simulink subsystem "PvtSubSys_LATC"  (R2020b)
settings: Solver=VariableStepAuto  StartTime=0.0  StopTime=10.0  RelTol=1e-3
values from neighbouring files (symbols this model uses):
  P_Global_CharSpd_ms : value not decoded    [PubParsGlobal.sldd]
  P_Global_SteeringAngleRatio : value not decoded    [PubParsGlobal.sldd]
  P_Global_WheelBase_m : value not decoded    [PubParsGlobal.sldd]
  P_LCS_A0_Dis_BP : value not decoded    [SubMdlDD_LATC.sldd]
  P_LCS_A2_Curve_BP : value not decoded    [SubMdlDD_LATC.sldd]
  P_LCS_A2_LatAcc_BP : value not decoded    [SubMdlDD_LATC.sldd]
  P_LCS_A2_Pretime = 0.075    [SubMdlDD_LATC.sldd]
  P_LCS_A2S_FliterTime = 0.5    [SubMdlDD_LATC.sldd]
  P_LCS_AngErrReversSign_SourceSW = 1.0    [SubMdlDD_LATC.sldd]
  P_LCS_AngleErrorReversTorq : value not decoded    [SubMdlDD_LATC.sldd]
  P_LCS_AngleErrorReversTorq_LC_TarAngleBp : value not decoded    [SubMdlDD_LATC.sldd]
  P_LCS_AngleErrorReversTorq_LC_TarAngleFac : value not decoded    [SubMdlDD_LATC.sldd]
  P_LCS_AngleErrorReversTorq_LC_VehSpdBp : value not decoded    [SubMdlDD_LATC.sldd]
  P_LCS_AngleErrorReversTorq_LC_VehSpdVal : value not decoded    [SubMdlDD_LATC.sldd]
  P_LCS_AngleErrorReversTorq_VehSpdBp : value not decoded    [SubMdlDD_LATC.sldd]
  P_LCS_AngleErrorReversTorq_VehSpdFac : value not decoded    [SubMdlDD_LATC.sldd]
  P_LCS_AngleFilterTime = 0.1    [SubMdlDD_LATC.sldd]
  P_LCS_AngleSlope_AES_Active = 0.4 0.4 0.4 0.35 0.35 0.35 0.35 0.35 0.35 0.3 0.3 0.3 0.3 0.3 0.3 0.3 0.3 0.3 0.3 0.4 0.4 0.4 0.35 0.35 0.35 0.35 0.35 0.35 0.3 0.3 0.3 0.3 0.3 0.3 0.3 0.3 0.3 0.3 0.4 0.4 0.4 0.35 0.35 0.35 0.35 0.35 0.35 0.3 0.3 0.3 0.3 0.3 0.3 0.3 0.3 0.3 0.3 0.4 0.4 0.4 0.35 0.35 0.35 0.35 0.35 0.35 0.3 0.3 0.3 0.3 0.3 0.3 0.3 0.3 0.3 0.3 0.4 0.4 0.4 0.35 0.35 0.35 0.35 0.35 0.35 0.3 0.3 0.3 0.3 0.3 0.3 0.3 0.    [SubMdlDD_LATC.sldd]
  P_LCS_AngleSlope_ESS_Add = 1.0 1.0 1.0 1.0 2.0 2.0 2.0 7.0 7.0 7.0 7.0 7.0 7.0 7.0 7.0 7.0 7.0 7.0 7.0 1.0 1.0 1.0 1.0 2.0 2.0 2.0 7.0 7.0 7.0 7.0 7.0 7.0 7.0 7.0 7.0 7.0 7.0 7.0 1.0 1.0 1.0 1.0 2.0 2.0 2.0 7.0 7.0 7.0 7.0 7.0 7.0 7.0 7.0 7.0 7.0 7.0 7.0 1.0 1.0 1.0 1.0 2.0 2.0 2.0 7.0 7.0 7.0 7.0 7.0 7.0 7.0 7.0 7.0 7.0 7.0 7.0 1.0 1.0 1.0 1.0 7.5 7.5 7.5 7.5 7.5 7.5 7.5 7.5 7.5 7.5 7.5 8.0 8.0 8.0 8.0 1.0 1.0 1.0 1.0 7.5    [SubMdlDD_LATC.sldd]
  P_LCS_AngleSlope_LC_Eco = 0.4 0.4 0.4 0.35 0.35 0.35 0.35 0.35 0.35 0.3 0.3 0.3 0.3 0.3 0.3 0.3 0.3 0.3 0.3 0.4 0.4 0.4 0.35 0.35 0.35 0.35 0.35 0.35 0.3 0.3 0.3 0.3 0.3 0.3 0.3 0.3 0.3 0.3 0.4 0.4 0.4 0.35 0.35 0.35 0.35 0.35 0.35 0.3 0.3 0.3 0.3 0.3 0.3 0.3 0.3 0.3 0.3 0.4 0.4 0.4 0.35 0.35 0.35 0.35 0.35 0.35 0.3 0.3 0.3 0.3 0.3 0.3 0.3 0.3 0.3 0.3 0.4 0.4 0.4 0.35 0.35 0.35 0.35 0.35 0.35 0.3 0.3 0.3 0.3 0.3 0.3 0.3 0.    [SubMdlDD_LATC.sldd]
  P_LCS_AngleSlope_LC_Nomal = 0.4 0.4 0.4 0.35 0.35 0.35 0.35 0.35 0.35 0.3 0.3 0.3 0.3 0.3 0.3 0.3 0.3 0.3 0.3 0.4 0.4 0.4 0.35 0.35 0.35 0.35 0.35 0.35 0.3 0.3 0.3 0.3 0.3 0.3 0.3 0.3 0.3 0.3 0.4 0.4 0.4 0.35 0.35 0.35 0.35 0.35 0.35 0.3 0.3 0.3 0.3 0.3 0.3 0.3 0.3 0.3 0.3 0.4 0.4 0.4 0.35 0.35 0.35 0.35 0.35 0.35 0.3 0.3 0.3 0.3 0.3 0.3 0.3 0.3 0.3 0.3 0.4 0.4 0.4 0.35 0.35 0.35 0.35 0.35 0.35 0.3 0.3 0.3 0.3 0.3 0.3 0.3 0.    [SubMdlDD_LATC.sldd]
  P_LCS_AngleSlope_LC_Sport = 0.4 0.4 0.4 0.35 0.35 0.35 0.35 0.35 0.35 0.3 0.3 0.3 0.3 0.3 0.3 0.3 0.3 0.3 0.3 0.4 0.4 0.4 0.35 0.35 0.35 0.35 0.35 0.35 0.3 0.3 0.3 0.3 0.3 0.3 0.3 0.3 0.3 0.3 0.4 0.4 0.4 0.35 0.35 0.35 0.35 0.35 0.35 0.3 0.3 0.3 0.3 0.3 0.3 0.3 0.3 0.3 0.3 0.4 0.4 0.4 0.35 0.35 0.35 0.35 0.35 0.35 0.3 0.3 0.3 0.3 0.3 0.3 0.3 0.3 0.3 0.3 0.4 0.4 0.4 0.35 0.35 0.35 0.35 0.35 0.35 0.3 0.3 0.3 0.3 0.3 0.3 0.3 0.    [SubMdlDD_LATC.sldd]
  P_LCS_AngleSlope_LCK = 0.4 0.4 0.4 0.4 0.4 0.4 0.4 0.4 0.4 0.4 0.4 0.4 0.4 0.4 0.4 0.4 0.4 0.4 0.4 0.4 0.4 0.4 0.4 0.4 0.4 0.4 0.4 0.4 0.4 0.4 0.4 0.4 0.4 0.4 0.4 0.4 0.4 0.4 0.4 0.4 0.4 0.4 0.4 0.4 0.4 0.4 0.4 0.4 0.4 0.4 0.4 0.4 0.4 0.4 0.4 0.4 0.4 0.4 0.4 0.4 0.4 0.4 0.4 0.4 0.4 0.4 0.4 0.4 0.4 0.4 0.4 0.4 0.4 0.4 0.4 0.4 0.4 0.4 0.4 0.4 0.4 0.4 0.4 0.4 0.4 0.4 0.4 0.4 0.4 0.4 0.4 0.4 0.4 0.4 0.4 0.4 0.4 0.4 0.4 0.4    [SubMdlDD_LATC.sldd]
  P_LCS_AngleSlope_LCKIE = 0.4 0.4 0.4 0.4 0.4 0.4 0.4 0.4 0.4 0.4 0.4 0.4 0.4 0.4 0.4 0.4 0.4 0.4 0.4 0.4 0.4 0.4 0.4 0.4 0.4 0.4 0.4 0.4 0.4 0.4 0.4 0.4 0.4 0.4 0.4 0.4 0.4 0.4 0.4 0.4 0.4 0.4 0.4 0.4 0.4 0.4 0.4 0.4 0.4 0.4 0.4 0.4 0.4 0.4 0.4 0.4 0.4 0.4 0.4 0.4 0.4 0.4 0.4 0.4 0.4 0.4 0.4 0.4 0.4 0.4 0.4 0.4 0.4 0.4 0.4 0.4 0.4 0.4 0.4 0.4 0.4 0.4 0.4 0.4 0.4 0.4 0.4 0.4 0.4 0.4 0.4 0.4 0.4 0.4 0.4 0.4 0.4 0.4 0.4 0.4    [SubMdlDD_LATC.sldd]
  P_LCS_AngleSlope_LKA = 0.2 0.2 0.3 0.4 0.4 0.4 0.4 0.4 0.4 0.4 0.4 0.4 0.4 0.4 0.4 0.4 0.4 0.4 0.4 0.2 0.2 0.3 0.4 0.4 0.4 0.4 0.4 0.4 0.4 0.4 0.4 0.4 0.4 0.4 0.4 0.4 0.4 0.4 0.2 0.2 0.3 0.4 0.4 0.4 0.4 0.4 0.4 0.4 0.4 0.4 0.4 0.4 0.4 0.4 0.4 0.4 0.4 0.2 0.2 0.3 0.4 0.4 0.4 0.4 0.4 0.4 0.4 0.4 0.4 0.4 0.4 0.4 0.4 0.4 0.4 0.4 0.2 0.2 0.3 0.4 0.4 0.4 0.4 0.4 0.4 0.4 0.4 0.4 0.4 0.4 0.4 0.4 0.4 0.4 0.4 0.2 0.2 0.3 0.4 0.4    [SubMdlDD_LATC.sldd]
  P_LCS_AngleSlope_Spd_BP : value not decoded    [SubMdlDD_LATC.sldd]
  P_LCS_CurAngleFiltEnable = 1    [SubMdlDD_LATC.sldd]
  P_LCS_CurAngleFilterFC = 2.0    [SubMdlDD_LATC.sldd]
  P_LCS_CurentOffset_LimitValue = 0.001    [SubMdlDD_LATC.sldd]
  P_LCS_CurOffset_SterAngleSpd_Enable = 0.0    [SubMdlDD_LATC.sldd]
  P_LCS_CurOffset_SterAngleSpd_LimitValue = 6.0    [SubMdlDD_LATC.sldd]
  P_LCS_CurOffset_VehicleSpd_LimitValue = 7.0    [SubMdlDD_LATC.sldd]
  P_LCS_CurOffsetA2_Enable = 0.0    [SubMdlDD_LATC.sldd]
  P_LCS_CurOffsetA2_FliterTime = 0.2    [SubMdlDD_LATC.sldd]
  P_LCS_DeltaEps_SpdBp : value not decoded    [SubMdlDD_LATC.sldd]
  P_LCS_DeltaEps_TimeVal : value not decoded    [SubMdlDD_LATC.sldd]
  P_LCS_DesAngle_DelaySample : value not decoded    [SubMdlDD_LATC.sldd]
  P_LCS_DetNoOverRide_DrvTrq_TH : value not decoded    [SubMdlDD_LATC.sldd]
  P_LCS_DetOverRide_DrvTrq_TH : value not decoded    [SubMdlDD_LATC.sldd]
  P_LCS_EPSNotActiveSpdValue = 3.0    [SubMdlDD_LATC.sldd]
  P_LCS_ESS_AngleSlope_Limit = 2.9    [SubMdlDD_LATC.sldd]
  P_LCS_ESS_LogicTest_Enable = 1.0    [SubMdlDD_LATC.sldd]
  P_LCS_ESS_MaxTorqSlope : value not decoded    [SubMdlDD_LATC.sldd]
  P_LCS_ESS_NotActiveFlgDelayTime = 0.0    [SubMdlDD_LATC.sldd]
  P_LCS_ESS_NotActiveFlgDelayTimeSW = 0.0    [SubMdlDD_LATC.sldd]
  P_LCS_ESS_SteerAngleErr : value not decoded    [SubMdlDD_LATC.sldd]
  P_LCS_ESS_SteerAngleFilterTime = 0.2    [SubMdlDD_LATC.sldd]
  P_LCS_ESS_TarAngleFilterTime = 0.2    [SubMdlDD_LATC.sldd]
  P_LCS_ESSAngleSW2 = 0.0    [SubMdlDD_LATC.sldd]
  P_LCS_ESSOverrideTime1 = 0.06    [SubMdlDD_LATC.sldd]
  P_LCS_ESSOverrideTime2 = 0.06    [SubMdlDD_LATC.sldd]
  P_LCS_ESSOverrideTime3 = 0.06    [SubMdlDD_LATC.sldd]
  P_LCS_ESSOverrideValue1 = 20.0    [SubMdlDD_LATC.sldd]
  P_LCS_ESSOverrideValue2 = 20.0    [SubMdlDD_LATC.sldd]
  P_LCS_FF_A0_Speed_Factor : value not decoded    [SubMdlDD_LATC.sldd]
  P_LCS_FF_A0_Torq : value not decoded    [SubMdlDD_LATC.sldd]
  P_LCS_FF_EnableSpd = 5.0    [SubMdlDD_LATC.sldd]
  P_LCS_FF_LCRevs_SpdBP : value not decoded    [SubMdlDD_LATC.sldd]
  P_LCS_FF_LCRevs_SpdVal : value not decoded    [SubMdlDD_LATC.sldd]
  P_LCS_FF_LCRevs_TimeBP : value not decoded    [SubMdlDD_LATC.sldd]
  P_LCS_FF_LCRevs_TimeFacVal : value not decoded    [SubMdlDD_LATC.sldd]
  P_LCS_FF_Param_CurveBp : value not decoded    [SubMdlDD_LATC.sldd]
  P_LCS_FF_Param_CurveFac : value not decoded    [SubMdlDD_LATC.sldd]
  P_LCS_FF_Speed_Bp : value not decoded    [SubMdlDD_LATC.sldd]
  P_LCS_FF_Speed_Factor : value not decoded    [SubMdlDD_LATC.sldd]
  P_LCS_FF_TarAngleTorq_Bp : value not decoded    [SubMdlDD_LATC.sldd]
  P_LCS_FF_TarAngleTorq_Factor : value not decoded    [SubMdlDD_LATC.sldd]
  P_LCS_FFW_Torq_AngleBp : value not decoded    [SubMdlDD_LATC.sldd]
  P_LCS_FFW_Torq_SpdBp : value not decoded    [SubMdlDD_LATC.sldd]
  P_LCS_FFW_Torq_V71 : value not decoded    [SubMdlDD_LATC.sldd]
  P_LCS_FFWSwitch : value not decoded    [SubMdlDD_LATC.sldd]
  P_LCS_IN_Offset_Test_SW = 0.0    [SubMdlDD_LATC.sldd]
  P_LCS_IN_Offset_Test_Value = 0.0    [SubMdlDD_LATC.sldd]
  P_LCS_LatAcc2CurveSW = 0.0    [SubMdlDD_LATC.sldd]
  P_LCS_LC_Complete_PreDisFac : value not decoded    [SubMdlDD_LATC.sldd]
  P_LCS_LCK_preDis_Nomal : value not decoded    [SubMdlDD_LATC.sldd]
  P_LCS_MaxTorqSlope : value not decoded    [SubMdlDD_LATC.sldd]
  P_LCS_NoOverRideTime_TH_s : value not decoded    [SubMdlDD_LATC.sldd]
  P_LCS_Offset_FliterTime = 2.0    [SubMdlDD_LATC.sldd]
  P_LCS_OverRideDetect_enable : value not decoded    [SubMdlDD_LATC.sldd]
  P_LCS_OverRideTime_TH_s : value not decoded    [SubMdlDD_LATC.sldd]
  P_LCS_PID_A0_BP : value not decoded    [SubMdlDD_LATC.sldd]
  P_LCS_PID_A0_FF_SW = 0.0    [SubMdlDD_LATC.sldd]
  P_LCS_PID_A0_P : value not decoded    [SubMdlDD_LATC.sldd]
  P_LCS_PID_AngErrFacBp : value not decoded    [SubMdlDD_LATC.sldd]
  P_LCS_PID_AngErrFacBp_P : value not decoded    [SubMdlDD_LATC.sldd]
  P_LCS_PID_AngErrFacVal : value not decoded    [SubMdlDD_LATC.sldd]
  P_LCS_PID_AngErrFacVal_P : value not decoded    [SubMdlDD_LATC.sldd]
  P_LCS_PID_DisableKi_CurveVal = 0.003    [SubMdlDD_LATC.sldd]
  P_LCS_PID_DrvTorqFacBp : value not decoded    [SubMdlDD_LATC.sldd]
  P_LCS_PID_DrvTorqFacVal : value not decoded    [SubMdlDD_LATC.sldd]
  P_LCS_PID_Ki_TarAng_ESS : value not decoded    [SubMdlDD_LATC.sldd]
  P_LCS_PID_Kp_TarAng_ESS : value not decoded    [SubMdlDD_LATC.sldd]
  P_LCS_PID_Kp_TarAng_ESS2 : value not decoded    [SubMdlDD_LATC.sldd]
  P_LCS_PID_Kp_TarTorq_ESS : value not decoded    [SubMdlDD_LATC.sldd]
  P_LCS_PID_Param_CurveBp : value not decoded    [SubMdlDD_LATC.sldd]
  P_LCS_PID_Param_CurveFac : value not decoded    [SubMdlDD_LATC.sldd]
  P_LCS_PID_Param_GainSwitch : value not decoded    [SubMdlDD_LATC.sldd]
  P_LCS_PID_Param_Kd : value not decoded    [SubMdlDD_LATC.sldd]
  P_LCS_PID_Param_KdFilterTime : value not decoded    [SubMdlDD_LATC.sldd]
  P_LCS_PID_Param_Ki : value not decoded    [SubMdlDD_LATC.sldd]
  P_LCS_PID_Param_KiFreaseWhenLC_Enable : value not decoded    [SubMdlDD_LATC.sldd]
  P_LCS_PID_Param_Kp : value not decoded    [SubMdlDD_LATC.sldd]
  P_LCS_PID_Param_Speed_Adapt : value not decoded    [SubMdlDD_LATC.sldd]
  P_LCS_PID_Param_Speed_Factor_D : value not decoded    [SubMdlDD_LATC.sldd]
  P_LCS_PID_Param_Speed_Factor_I : value not decoded    [SubMdlDD_LATC.sldd]
  P_LCS_PID_Param_Speed_Factor_P : value not decoded    [SubMdlDD_LATC.sldd]
  P_LCS_PID_Param_SteerWheelAngle_Adapt : value not decoded    [SubMdlDD_LATC.sldd]
  P_LCS_PID_Param_SteerWheelAngle_Factor_D : value not decoded    [SubMdlDD_LATC.sldd]
  P_LCS_PID_Param_SteerWheelAngle_Factor_P : value not decoded    [SubMdlDD_LATC.sldd]
  P_LCS_PID_Param_SteerWheelSpd_Adapt : value not decoded    [SubMdlDD_LATC.sldd]
  P_LCS_PID_Param_SteerWheelSpd_Factor_D : value not decoded    [SubMdlDD_LATC.sldd]
  P_LCS_PID_Param_SteerWheelSpd_Factor_P : value not decoded    [SubMdlDD_LATC.sldd]
  P_LCS_PID_SteerAngSpdLim : value not decoded    [SubMdlDD_LATC.sldd]
  P_LCS_preDis_AES_Fac = 0.0 0.0 0.0 0.0 -0.1 -0.1 -0.1 -0.1 -0.1 -0.1 0.1 0.1 0.1 0.2 0.2 0.2 0.2 0.2 0.2 0.0 0.0 0.0 0.0 -0.1 -0.1 -0.1 -0.1 -0.1 -0.1 0.1 0.1 0.1 0.2 0.2 0.2 0.2 0.2 0.2 0.0 0.0 0.0 0.0 -0.1 -0.1 -0.1 -0.1 -0.1 -0.1 0.1 0.1 0.1 0.2 0.2 0.2 0.2 0.2 0.2 0.0 0.0 0.0 0.0 -0.1 -0.1 -0.1 -0.1 -0.1 -0.1 0.1 0.1 0.1 0.2 0.2 0.2 0.2 0.2 0.2 0.0 0.0 0.0 0.0 -0.1 -0.1 -0.1 -0.1 -0.1 -0.1 0.2 0.2 0.2 0.35 0.35 0.35    [SubMdlDD_LATC.sldd]
  P_LCS_preDis_LC_Eco_Fac = 0.0 0.0 0.0 0.0 0.25 0.3 0.3 0.3 0.35 0.35 0.45 0.45 0.45 0.55 0.55 0.55 0.55 0.55 0.55 0.0 0.0 0.0 0.0 0.25 0.3 0.3 0.3 0.35 0.35 0.45 0.45 0.45 0.55 0.55 0.55 0.55 0.55 0.55 0.0 0.0 0.0 0.0 0.25 0.3 0.3 0.3 0.35 0.35 0.45 0.45 0.45 0.55 0.55 0.55 0.55 0.55 0.55 0.0 0.0 0.0 0.0 0.25 0.3 0.3 0.3 0.35 0.35 0.45 0.45 0.45 0.55 0.55 0.55 0.55 0.55 0.55 0.0 0.0 0.0 0.0 0.25 0.3 0.3 0.3 0.35 0.35 0.55    [SubMdlDD_LATC.sldd]
  P_LCS_preDis_LC_Fac = 0.0 0.0 0.0 0.0 -0.1 -0.1 -0.1 -0.1 -0.1 -0.1 0.1 0.1 0.1 0.2 0.2 0.2 0.2 0.2 0.2 0.0 0.0 0.0 0.0 -0.1 -0.1 -0.1 -0.1 -0.1 -0.1 0.1 0.1 0.1 0.2 0.2 0.2 0.2 0.2 0.2 0.0 0.0 0.0 0.0 -0.1 -0.1 -0.1 -0.1 -0.1 -0.1 0.1 0.1 0.1 0.2 0.2 0.2 0.2 0.2 0.2 0.0 0.0 0.0 0.0 -0.1 -0.1 -0.1 -0.1 -0.1 -0.1 0.1 0.1 0.1 0.2 0.2 0.2 0.2 0.2 0.2 0.0 0.0 0.0 0.0 -0.1 -0.1 -0.1 -0.1 -0.1 -0.1 0.2 0.2 0.2 0.35 0.35 0.35    [SubMdlDD_LATC.sldd]
  P_LCS_preDis_LC_Nomal_Fac = 0.0 0.0 0.0 0.0 -0.1 -0.1 -0.1 -0.1 -0.1 -0.1 0.1 0.1 0.1 0.2 0.2 0.2 0.2 0.2 0.2 0.0 0.0 0.0 0.0 -0.1 -0.1 -0.1 -0.1 -0.1 -0.1 0.1 0.1 0.1 0.2 0.2 0.2 0.2 0.2 0.2 0.0 0.0 0.0 0.0 -0.1 -0.1 -0.1 -0.1 -0.1 -0.1 0.1 0.1 0.1 0.2 0.2 0.2 0.2 0.2 0.2 0.0 0.0 0.0 0.0 -0.1 -0.1 -0.1 -0.1 -0.1 -0.1 0.1 0.1 0.1 0.2 0.2 0.2 0.2 0.2 0.2 0.0 0.0 0.0 0.0 -0.1 -0.1 -0.1 -0.1 -0.1 -0.1 0.2 0.2 0.2 0.35 0.35 0.35    [SubMdlDD_LATC.sldd]
  P_LCS_preDis_LC_Sport_Fac = 0.0 0.0 0.0 0.0 -0.1 -0.1 -0.1 -0.1 -0.1 -0.1 0.1 0.1 0.1 0.2 0.2 0.2 0.2 0.2 0.2 0.0 0.0 0.0 0.0 -0.1 -0.1 -0.1 -0.1 -0.1 -0.1 0.1 0.1 0.1 0.2 0.2 0.2 0.2 0.2 0.2 0.0 0.0 0.0 0.0 -0.1 -0.1 -0.1 -0.1 -0.1 -0.1 0.1 0.1 0.1 0.2 0.2 0.2 0.2 0.2 0.2 0.0 0.0 0.0 0.0 -0.1 -0.1 -0.1 -0.1 -0.1 -0.1 0.1 0.1 0.1 0.2 0.2 0.2 0.2 0.2 0.2 0.0 0.0 0.0 0.0 -0.1 -0.1 -0.1 -0.1 -0.1 -0.1 0.2 0.2 0.2 0.35 0.35 0.35    [SubMdlDD_LATC.sldd]
  P_LCS_preDis_LCK_A2Curve_Fac2 : value not decoded    [SubMdlDD_LATC.sldd]
  ... (+20 more)
undefined symbols (not defined in the file or in its folder): P_LCS_A2_CurrentOffsetFliterTime, P_LCS_AngleSlope_ELK, P_LCS_AngleSlope_ESS, P_LCS_AngleSlope_LC_Cancel, P_LCS_AngleSlope_LCK_Curve_Fac, P_LCS_CurSteerAngleOffsetLimit_Low, P_LCS_CurSteerAngleOffsetLimit_Up, P_LCS_DesLaneA0, P_LCS_DesLaneA1, P_LCS_ESS_preDis_Nomal, P_LCS_ESSAngleSW, P_LCS_ESSAngSlope_SW, P_LCS_LATC_Effect, P_LCS_MinTorqSlope, P_LCS_PID_Param_Kifactor, P_LCS_preDis_ELK_Fac, P_LCS_preDis_ESS_Fac, P_LCS_preDis_LCK_A2Curve_Fac, P_LCS_preDis_LCK_Fac, P_LCS_StateActiv_AngleSlope, P_LCS_StateActiveFlg_BP, P_LCS_TorqSlope_AngleErrorBp, P_LCS_TorqSlope_AngleErrorVal, P_LCS_TorqSlope_AngleSpdBp, P_LCS_TorqSlope_AngleSpdVal, P_LCS_TorqSlope_TorqErrorBp, P_LCS_TorqSlope_TorqErrorVal
libraries: simulink x59
(part 6 of 75)

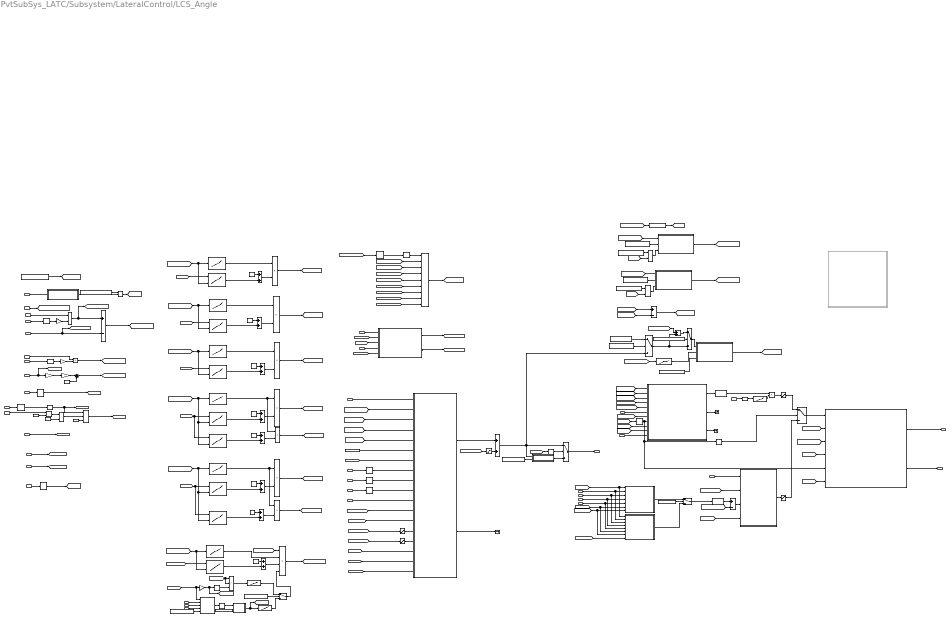
== system PvtSubSys_LATC/Subsystem/LateralControl/LCS_Angle ==
  note: 0:No Function Active
      | 1:LCK Active
      | 2:LCKIE Active
      | 3:LC Normal Active
      | 4:LKA Active
      | 5:ELK Active
      | 6:ESS Active
      | 7:LC Eco Active
      | 8:LC Sport Active
      | 9:LC cancel
      | 10: AES Active
  note: ESS_AES
  note: ELK && LC
  note: Steer Wheel Angle Slope Manage
  note: LCK_LKA_LCKIE_Normal
  note: Sport
  note: Eco
  note: Normal
  note: PreDis_Manage
  note: Torque
  note: 0:No Function Active
      | 1:LCK Active
      | 2:LCKIE Active
      | 3:LC Normal Active
      | 4:LKA Active
      | 5:ELK Active
      | 6:ESS AES Active
      | 7:LC Eco Active
      | 8:LC Sport Active
  note: 模型变更记录
      | 2021/05/31 修改PreDis观测量、增加PreDisFac观测量；（版本：36010506）
      | 2021/06/02 增加弯道关于A2的PreDisFac标定量；（版本：36010506）
      | 2021/06/08 按A0 = 0.8m退出LC修改三种换道预瞄距离系数；增加LCS_EpsTrqReqValue、LCS_EpsTrqReqValueVld观测量（版本：36010506）
      | 2021/06/17 增加单独的ELK、ESSAES预瞄距离参数表；增加LCS_LC_ESSPredis、LCS_LC_ELKPredis观测量；增加ESS、ELS手动调试开关（版本：36170507）
      | 修改LCS模型输出观测量命名，例：LCS_ReqEPSTrgAngle -> LCS_OUT_ReqEPSTrgAngle
      | 2021/07/05 更新ELK标定参数（版本：37050508）
      | 2021/07/12 更新P_LCS_preDis_LCK_A2Curve_Fac标定参数（版本：37120509）
      | 2021/07/15 增加弯道内通过预瞄曲率查表LCK_Predis的Fac修正系数逻辑（版本：37120509）
      | 2021/07/20 增加换道取消P_LCS_preDis_LC_Fac修正系数（版本：37120509）
      | 2021/08/03 增加ESS请求角度斜率限制，防止EPS故障（版本：37120509）
      | 2021/08/04 增加EPS转速>150，ESS退出逻辑，暂用于测试，后期可能会删除（版本：37120509）
      | 2021/08/04 P_LCS_LatAcc2CurveSW设置默认为0
      | 2021/08/09 增加ESS测试逻辑，暂时测试版
      | 2021/08/16 ESS标定数据更改、增加转角与扭矩得ESS开关
      | 2021/08/20 A2项逻辑默认开，LCK_Fac全部置0，P_LCS_preDis_LCK_A2Curve_Fac2参数置：1 1 1 0.85 0.75 0.6 0.5 0.3 0.3 0.25
      | 2021/08/21 修改5kph以下LineValid置零逻辑（版本：38210511）
      | 2021/08/23 修改5kph以下LineValid置零，置零后目标角度不滤波（版本：38210511）
      | 2021/08/23 修改LC换道取消逻辑和标定参数（版本：38230512）
      | 2021/08/24 ESS最初为~=6，因测试出当DangerLevel==6时，状态可能跳变的问题。改成<=5，避免数据类型导致数据比较出现的问题
      | 2021/08/24 增加EPS故障监控逻辑、PID中FF和Kp增加A0项（版本：38240513）
      | 2021/08/25 修改AngleErrorRevers反向符号逻辑（版本：38250514）
      | 2021/08/30 模型整理（版本：38300515）
      | 2021/09/07 修改ESS置位条件（版本：39070516）
      | 2021/09/15 增加port口描述及接口数据类型（版本：39150517）
      | 2021/10/18 LineValid置零逻辑阈值由5kph->3kph;同步CurrentOffset激活逻辑;增加换道超调控制逻辑(默认关闭)（版本：10180518）
      | 2021/10/20 修改内部CurrentOffset激活条件，改成根据曲率进行滤波（版本：10200519)
      | 2021/11/01 增加大框接口LATC_Effect（版本：11010520)
      | 2021/11/03 增加依据曲率修正LCK的AngelSlope（版本：11030521)
      | 2021/11/04 增加内部CurrentOffset计算限值（版本：11040522)
      | 2021/11/08 修改内部CurrentOffset根据曲率进行滤波的时间（版本：11080523)
  note: ESS请求角度斜率限制，防止EPS故障
  note: 最初为~=6，因测试出当DangerLevel==6时，状态可能跳变的问题。改成<=5避免数据类型导致数据比较出现的问题
  canSteerWheelAngle : Inport
  canSteerWheelAngleSign : Inport  Port=2
  canEPS_LKATorqOvrlDlvd : Inport  Port=3
  canEPS_DrvInputTorq : Inport  Port=4
  canSteerWheelSpd : Inport  Port=5
  canSteerWheelSpdSign : Inport  Port=6
  SteerAngleOffset_deg : Inport  Port=7
  eviVxvRef_ms : Inport  Port=8
  desLaneValid : Inport  Port=9
  desLaneA3 : Inport  Port=10  OutDataTypeStr=single
  desLaneA2 : Inport  Port=11
  desLaneA1 : Inport  Port=12
  desLaneA0 : Inport  Port=13
  TarDangerlLevel : Inport  Port=14
  kapTraj1 : Inport  Port=15
  CurrentSteerAngleOffset : Inport  Port=16
  LaneWidth : Inport  Port=17
  2-D Lookup Table1 : Lookup_n-D  BreakpointsForDimension1=P_LCS_A0_Dis_BP  BreakpointsForDimension2=P_LCS_preDis_spd  Table=P_LCS_preDis_LC_Nomal_Fac  ExtrapMethod=Clip  UseLastTableValue=on  InternalRulePriority=Speed  RndMeth=Simplest  InputSameDT=on
      settings: InputPortMap=u0,u1
  2-D Lookup Table2 : Lookup_n-D  BreakpointsForDimension1=P_LCS_A0_Dis_BP  BreakpointsForDimension2=P_LCS_preDis_spd  Table=P_LCS_preDis_LCK_Fac  ExtrapMethod=Clip  UseLastTableValue=on  InternalRulePriority=Speed  RndMeth=Simplest  InputSameDT=on
      settings: InputPortMap=u0,u1
  Abs{1..4} (4 alike) : Abs
  Add : Sum  Inputs=+-
  Add1 : Sum  Inputs=+-
  Add{2,4..5,7..12} (9 alike) : Sum
  Add3 : Sum  Inputs=+-
  Add6 : Sum  AccumDataTypeStr=single
  AngSlopeCalc : Subsystem
  Bias1 : Bias  Bias=-0.5
  Bias2 : Bias  Bias=-0.5
  Compare To Constant : simulink/Logic and Bit Operations/Compare To Constant  relop=~=  const=6  OutDataTypeStr=boolean
  Compare To Constant1 : simulink/Logic and Bit Operations/Compare To Constant  relop=~=  const=6  OutDataTypeStr=boolean
  Compare To Constant3 : simulink/Logic and Bit Operations/Compare To Constant  relop=<=  const=57  OutDataTypeStr=boolean
  Constant : Constant  Value=P_Global_SteeringAngleRatio  OutDataTypeStr=double
  Constant1 : Constant  Value=1000  OutDataTypeStr=single
  Constant10 : Constant  Value=P_LCS_CurAngleFiltEnable
  Constant11 : Constant  Value=P_LCS_TarAngleFilterEnable
  Constant{12..14,17..18,22,24,26} (8 alike) : Constant  OutDataTypeStr=single
  Constant15 : Constant  Value=P_LCS_OverRideDetect_enable
  Constant16 : Constant  Value=P_LCS_ESS_AngleSlope_Limit  OutDataTypeStr=single
  Constant2 : Constant  Value=P_LCS_LatAcc2CurveSW
  Constant20 : Constant  Value=P_LCS_A2S_FliterTime
  Constant21 : Constant  Value=P_LCS_A2_Pretime  OutDataTypeStr=single
  Constant4 : Constant  Value=3.6  OutDataTypeStr=single
  Constant5 : Constant  Value=P_LCS_SW
  Constant6 : Constant  Value=3  OutDataTypeStr=single
  Constant7 : Constant  Value=4  OutDataTypeStr=single
  Constant8 : Constant  Value=1.3  OutDataTypeStr=single
  Constant9 : Constant  Value=P_LCS_CurAngleFiltEnable
  Data Type Conversion : DataTypeConversion  OutDataTypeStr=single
  Data Type Conversion5 : DataTypeConversion  OutDataTypeStr=single
  Direct Lookup Table (n-D) : LookupNDDirect  NumberOfTableDimensions=1  Table=[4 4 4 1 4 5 6 2 3 7 8]  TableDataTypeStr=uint8
  Direct Lookup Table (n-D)1 : LookupNDDirect  NumberOfTableDimensions=1  Table=[0 1 2 3 4 5 6 3 3]  TableDataTypeStr=uint8
  Divide : Product  Inputs=**/
  Gain1 : Gain  Gain=2
  Gain2 : Gain  Gain=-2
  Gain3 : Gain  Gain=3.6
  Gain4 : Gain  Gain=1.03
  Gain5 : Gain  Gain=-2
  LCS_LC_ELK_preDis_TB : Lookup_n-D  BreakpointsForDimension1=P_LCS_A0_Dis_BP  BreakpointsForDimension2=P_LCS_preDis_spd  Table=P_LCS_preDis_ELK_Fac  ExtrapMethod=Clip  UseLastTableValue=on  InternalRulePriority=Speed  RndMeth=Simplest  InputSameDT=on
      settings: InputPortMap=u0,u1
  LCS_LC_ELK_preDis_TB1 : Lookup_n-D  BreakpointsForDimension1=P_LCS_A0_Dis_BP  BreakpointsForDimension2=P_LCS_preDis_spd  Table=P_LCS_preDis_LC_Fac  ExtrapMethod=Clip  UseLastTableValue=on  InternalRulePriority=Speed  RndMeth=Simplest  InputSameDT=on
      settings: InputPortMap=u0,u1
  LCS_LC_ESSAES_preDis_TB : Lookup_n-D  BreakpointsForDimension1=P_LCS_A0_Dis_BP  BreakpointsForDimension2=P_LCS_preDis_spd  Table=P_LCS_preDis_ESS_Fac  ExtrapMethod=Clip  UseLastTableValue=on  InternalRulePriority=Speed  RndMeth=Simplest  InputSameDT=on
      settings: InputPortMap=u0,u1
  LCS_LC_ESSAES_preDis_TB1 : Lookup_n-D  BreakpointsForDimension1=P_LCS_A0_Dis_BP  BreakpointsForDimension2=P_LCS_preDis_spd  Table=P_LCS_preDis_AES_Fac  ExtrapMethod=Clip  UseLastTableValue=on  InternalRulePriority=Speed  RndMeth=Simplest  InputSameDT=on
      settings: InputPortMap=u0,u1
  LCS_LC_Emergent_preDis_TB : Lookup_n-D  BreakpointsForDimension1=P_LCS_A0_Dis_BP  BreakpointsForDimension2=P_LCS_preDis_spd  Table=P_LCS_preDis_LC_Sport_Fac  ExtrapMethod=Clip  UseLastTableValue=on  InternalRulePriority=Speed  RndMeth=Simplest  InputSameDT=on
      settings: InputPortMap=u0,u1
  LC_Medium_preDis_Fac_TB : Lookup_n-D  BreakpointsForDimension1=P_LCS_A0_Dis_BP  BreakpointsForDimension2=P_LCS_preDis_spd  Table=P_LCS_preDis_LC_Eco_Fac  ExtrapMethod=Clip  UseLastTableValue=on  InternalRulePriority=Speed  RndMeth=Simplest  InputSameDT=on
      settings: InputPortMap=u0,u1
  LP filter : Subsystem
  LP filter1 : Subsystem
  LP filter2 : Subsystem
  LP filter3 : Subsystem
  Logical Operator1 : Logic  AllPortsSameDT=off  OutDataTypeStr=boolean
  Logical Operator2 : Logic  AllPortsSameDT=off  OutDataTypeStr=boolean
  Logical Operator3 : Logic  AllPortsSameDT=off  OutDataTypeStr=boolean
  MATLAB Function : MATLAB Function  TreatAsAtomicUnit=on
  MinMax : MinMax  Function=max  Inputs=2
  MinMax1 : MinMax  Inputs=2
  Multiport Switch4 : MultiPortSwitch  Inputs=8
  OverRideDetect : Subsystem
  PID1 : Subsystem
  Product{,3..9,12,15} (10 alike) : Product
  Product1 : Product  Inputs=3
  Product2 : Product  Inputs=4
  Saturation : Saturate  UpperLimit=10  LowerLimit=-10
  Saturation1 : Saturate  UpperLimit=10  LowerLimit=-10
  Saturation2 : Saturate  UpperLimit=10  LowerLimit=-10
  Saturation3 : Saturate  UpperLimit=P_LCS_TorqReqMax  LowerLimit=P_LCS_TorqReqMin  LinearizeAsGain=off
  Saturation4 : Saturate  UpperLimit=2.9  LowerLimit=-2.9  LinearizeAsGain=off
  Signal Copy{,1..6} (7 alike) : SignalConversion  OverrideOpt=off
  Subsystem : Subsystem
  Subsystem1 : Subsystem
  Subsystem2 : Subsystem
  Subsystem3 : Subsystem  Commented=on
  Subsystem4 : Subsystem
  Subsystem5 : Subsystem
  Sum : Sum  Inputs=|++
  Switch{,4..6} (4 alike) : Switch  Criteria=u2 ~= 0
  Switch1 : Switch  Criteria=u2 > Threshold
  Switch2 : Switch  Criteria=u2 > Threshold
  TarDangerlLevel2 : InportShadow  Port=14
  TargetSteerAngleCalc : Subsystem
  Terminator : Terminator
  Terminator1 : Terminator
  Terminator2 : Terminator
  TestAngleSwitch : Constant  Value=P_LCS_TestAngleSwitch
  TestAngleSwitch1 : Constant  Value=P_LCS_CurAngleFilterFC
  TestAngleSwitch2 : Constant  Value=P_LCS_TarAngleAddOffset_enable
  TestAngleSwitch3 : Constant  Value=P_LCS_CurAngleFilterFC
  TestTarAngle : Constant  Value=P_LCS_TestTarAngle
  canEPS_DrvInputTorq1 : InportShadow  Port=4
  canEPS_DrvInputTorq2 : InportShadow  Port=4
  canEPS_DrvInputTorq3 : InportShadow  Port=4
  desLaneA0_{1..4} (4 alike) : InportShadow  Port=13
  desLaneA1_1 : InportShadow  Port=12
  desLaneA1_4 : InportShadow  Port=12
  desLaneA2_2 : InportShadow  Port=11
  desLaneA2_3 : InportShadow  Port=11
  desLaneA3_2 : InportShadow  Port=10  OutDataTypeStr=single
  desLaneA3_4 : InportShadow  Port=10  OutDataTypeStr=single
  drvTorqIncFac : Lookup_n-D  NumberOfTableDimensions=1  BreakpointsForDimension1=P_LCS_PID_DrvTorqFacBp  Table=P_LCS_PID_DrvTorqFacVal  InternalRulePriority=Speed  RndMeth=Simplest  InputSameDT=on
  eviVxvRef_ms1 : InportShadow  Port=8
  eviVxvRef_ms6 : InportShadow  Port=8
  preDisMinTable1 : Lookup_n-D  NumberOfTableDimensions=1  BreakpointsForDimension1=P_LCS_TarAngleFilterFC_spdBp  Table=P_LCS_TarAngleFilterFC_spdVal  ExtrapMethod=Clip  InternalRulePriority=Speed  RndMeth=Simplest  InputSameDT=on
  preDisMin_TB : Lookup_n-D  NumberOfTableDimensions=1  BreakpointsForDimension1=P_LCS_preDis_spd  Table=P_LCS_LCK_preDis_Nomal  ExtrapMethod=Clip  InternalRulePriority=Speed  RndMeth=Simplest  InputSameDT=on
  preDisMin_TB1 : Lookup_n-D  NumberOfTableDimensions=1  BreakpointsForDimension1=P_LCS_preDis_spd  Table=P_LCS_LCK_preDis_Nomal  ExtrapMethod=Clip  InternalRulePriority=Speed  RndMeth=Simplest  InputSameDT=on
  preDisMin_TB2 : Lookup_n-D  NumberOfTableDimensions=1  BreakpointsForDimension1=P_LCS_preDis_spd  Table=P_LCS_LCK_preDis_Nomal  ExtrapMethod=Clip  UseLastTableValue=on  InternalRulePriority=Speed  RndMeth=Simplest  InputSameDT=on
  preDisMin_TB3 : Lookup_n-D  NumberOfTableDimensions=1  BreakpointsForDimension1=P_LCS_preDis_spd  Table=P_LCS_LCK_preDis_Nomal  ExtrapMethod=Clip  UseLastTableValue=on  InternalRulePriority=Speed  RndMeth=Simplest  InputSameDT=on
  preDisMin_TB4 : Lookup_n-D  NumberOfTableDimensions=1  BreakpointsForDimension1=P_LCS_preDis_spd  Table=P_LCS_LCK_preDis_Nomal  ExtrapMethod=Clip  InternalRulePriority=Speed  RndMeth=Simplest  InputSameDT=on
  preDisMin_TB5 : Lookup_n-D  NumberOfTableDimensions=1  BreakpointsForDimension1=P_LCS_preDis_spd  Table=P_LCS_ESS_preDis_Nomal  ExtrapMethod=Clip  InternalRulePriority=Speed  RndMeth=Simplest  InputSameDT=on
  predis_ayFac1 : Lookup_n-D  NumberOfTableDimensions=1  BreakpointsForDimension1=P_LCS_A2_Curve_BP  Table=P_LCS_preDis_LCK_A2Curve_Fac2  ExtrapMethod=Clip  UseLastTableValue=on  InternalRulePriority=Speed  RndMeth=Simplest  InputSameDT=on
  predis_ayFac4 : Lookup_n-D  NumberOfTableDimensions=1  BreakpointsForDimension1=P_LCS_A2_LatAcc_BP  Table=P_LCS_preDis_LCK_A2Curve_Fac  ExtrapMethod=Clip  UseLastTableValue=on  InternalRulePriority=Speed  RndMeth=Simplest  InputSameDT=on
  TrgSteerAngle : Outport  OutDataTypeStr=single
  epsTrqReqValue : Outport  Port=2
  epsTrqReqFlag : Outport  Port=3
  wires:
  [Predis_Curve] -> AngSlopeCalc/5(Predis_Curve)
  [LC_Complete_PreDisFac] -> Product2/1
  Signal Copy6/1 -> [TarDangerlLevel]  "LCS_IN_TarDangerlLevel"
  [TarDangerlLevel] -> Signal Copy/1
  [DisplaySpd_kph] -> TargetSteerAngleCalc/18(DisplaySpd_kph)
  [Eq_A0] -> TargetSteerAngleCalc/17(Eq_A0)
  [AES_PreDis] -> Multiport Switch4/9
  Product9/1 -> [AES_PreDis]  "LCS_LC_AESPredis"
  Add12/1 -> Product9/2
  LCS_LC_ESSAES_preDis_TB1/1 -> Add12/2  "LCS_LC_AESPredisFac"
  Constant17/1 -> Add12/1
  [TarDangerlLevel] -> TargetSteerAngleCalc/16(TarDangerlLevel)
  Constant16/1 -> Subsystem5/2(Slope)
  Subsystem5/1(out) -> Switch1/3
  Switch1/1 -> TrgSteerAngle/1  "LCS_OUT_ReqEPSTrgAngle"
  Compare To Constant1/1 -> Switch1/2
  [TarDangerlLevel] -> Compare To Constant1/1
  AngSlopeCalc/2(LC_Complete_PreDisFac) -> [LC_Complete_PreDisFac]  "LCS_LC_Complete_PreDisFac"
  [LC_PreDis] -> Multiport Switch4/8
  Product8/1 -> [LC_PreDis]  "LCS_LC_LCPredis"
  Add11/1 -> Product8/2
  LCS_LC_ELK_preDis_TB1/1 -> Add11/2  "LCS_LC_LCPredisFac"
  Constant18/1 -> Add11/1
  predis_ayFac1/1 -> Switch/3  "LCS_Predis_CurveFac"
  Switch/1 -> Product2/4  "LCS_LCK_CurveFac"
  LP filter/1(output) -> predis_ayFac1/1, [Predis_Curve]  "LCS_Predis_Curve"
  Constant2/1 -> Switch/2
  Constant20/1 -> LP filter/2(TorqFilterTime)
  Abs4/1 -> LP filter/1(Raw)
  MATLAB Function/1(PreCurve) -> Abs4/1
  Constant21/1 -> MATLAB Function/5(time)
  eviVxvRef_ms1/1 -> MATLAB Function/4(v)
  desLaneA3_4/1 -> MATLAB Function/3(c3)
  desLaneA1_4/1 -> MATLAB Function/2(c1)
  desLaneValid/1 -> Signal Copy4/1
  Signal Copy3/1 -> TargetSteerAngleCalc/10(A1)  "LCS_IN_desLaneA1"
  Signal Copy2/1 -> TargetSteerAngleCalc/9(A2)  "LCS_IN_desLaneA2"
  Signal Copy1/1 -> TargetSteerAngleCalc/8(A3)  "LCS_IN_desLaneA3"
  desLaneA0/1 -> Signal Copy5/1
  [ESS_PreDis] -> Multiport Switch4/7
  [ELK_PreDis] -> Multiport Switch4/6
  Product7/1 -> [ESS_PreDis]  "LCS_LC_ESSPredis"
  preDisMin_TB5/1 -> Product7/1, Product9/1
  Add10/1 -> Product7/2
  Constant13/1 -> Add10/1
  [DisplaySpd_kph] -> preDisMin_TB5/1, LCS_LC_ESSAES_preDis_TB/2, LCS_LC_ESSAES_preDis_TB1/2
  [Eq_A0] -> LCS_LC_ESSAES_preDis_TB/1, LCS_LC_ESSAES_preDis_TB1/1
  LCS_LC_ESSAES_preDis_TB/1 -> Add10/2  "LCS_LC_ESSPredisFac"
  LCS_LC_ELK_preDis_TB/1 -> Add9/2  "LCS_LC_ELKPredisFac"
  [Eq_A0] -> LCS_LC_ELK_preDis_TB/1, LCS_LC_ELK_preDis_TB1/1
  [DisplaySpd_kph] -> LCS_LC_ELK_preDis_TB/2, LCS_LC_ELK_preDis_TB1/2, preDisMin_TB4/1
  Constant12/1 -> Add9/1
  Add9/1 -> Product6/2
  preDisMin_TB4/1 -> Product6/1, Product8/1
  Product6/1 -> [ELK_PreDis]  "LCS_LC_ELKPredis"
  Subsystem4/3(sig_LCKTorq_PID_Torq) -> Terminator2/1
  Subsystem4/2(sig_LCKTorq_FF_Torq) -> Terminator1/1
  LP filter3/1(output) -> [SteerAngleSpdFilter_degs]  "LCS_SteerAngleSpdFilter_degs"
  LP filter2/1(output) -> [SteerAngleFilter_deg]  "LCS_SteerAngleFilter_deg"
  [DisplaySpd_kph] -> Compare To Constant3/1
  Compare To Constant3/1 -> [FilterEnable]
  TestAngleSwitch1/1 -> LP filter3/2(TorqFilterTime)
  Logical Operator2/1 -> LP filter3/3(enable)
  Constant9/1 -> Logical Operator2/1
  [FilterEnable] -> Logical Operator2/2
  [SteerAngleSpd_degs] -> LP filter3/1(Raw)
  [LCS_IN_SteerAngle_deg] -> LP filter2/1(Raw)
  TestAngleSwitch3/1 -> LP filter2/2(TorqFilterTime)
  Constant10/1 -> Logical Operator3/1
  [FilterEnable] -> Logical Operator3/2
  Logical Operator3/1 -> LP filter2/3(enable)
  LP filter1/1(output) -> [tarAngle]  "LCS_TarSteerAngle_deg"
  Constant11/1 -> LP filter1/3(enable)
  TestAngleSwitch2/1 -> Switch6/2
  TestTarAngle/1 -> Switch5/1
  TestAngleSwitch/1 -> Switch5/2
  Switch5/1 -> Switch6/3, Add4/2
  [DisplaySpd_kph] -> preDisMinTable1/1
  preDisMinTable1/1 -> LP filter1/2(TorqFilterTime)
  [SteerAngleOffset_deg] -> Add4/1
  Switch6/1 -> LP filter1/1(Raw)
  Add4/1 -> Switch6/1
  canEPS_DrvInputTorq3/1 -> Abs3/1
  Data Type Conversion/1 -> Product/1
  drvTorqIncFac/1 -> Product/2
  Abs3/1 -> drvTorqIncFac/1
  [Eq_A0] -> AngSlopeCalc/3(Eq_A0)
  Divide/1 -> [Eq_A0]  "LCS_EqA0"
  Constant7/1 -> MinMax1/2
  Constant6/1 -> MinMax/2
  MinMax/1 -> MinMax1/1
  MinMax1/1 -> Divide/2
  Constant4/1 -> Divide/3
  LaneWidth/1 -> MinMax/1
  [LCK_IE_LKA_Nomal_PreDis] -> Multiport Switch4/5
  [desLaneA0_abs] -> 2-D Lookup Table2/1
  [DisplaySpd_kph] -> 2-D Lookup Table2/2, preDisMin_TB3/1
  predis_ayFac4/1 -> Switch/1  "LCS_A2_LatAccFac"
  Constant14/1 -> Add2/1
  Add2/1 -> Product2/3
  [desLaneA2] -> Gain1/1, MATLAB Function/1(c2)  "LCS_IN_desLaneA2"
  Abs2/1 -> Product1/3
  Gain1/1 -> Abs2/1, [Curve]
  [vRef] -> Product1/2, Product1/1
  Product1/1 -> predis_ayFac4/1  "LCS_A2_LatAcc"
  preDisMin_TB3/1 -> Product2/2
  2-D Lookup Table2/1 -> Add2/2  "LCS_LCKPredisFac"
  Product2/1 -> [LCK_IE_LKA_Nomal_PreDis]  "LCS_LCKPredis"
  desLaneA0_2/1 -> AngSlopeCalc/4(desLane_A0)
  Multiport Switch4/1 -> [preDis]  "LCS_finalPredis"
  Direct Lookup Table (n-D)/1 -> Multiport Switch4/1  "LCS_LCType"
  AngSlopeCalc/1(AngSlope) -> [LCS_TarSteerAngleSlope]  "LCS_TarSteerAngleSlope"
  [Nomal_PreDis] -> Multiport Switch4/2
  [Eco_PreDis] -> Multiport Switch4/3
  [Sport_PreDis] -> Multiport Switch4/4
  Product15/1 -> [Sport_PreDis]  "LCS_LC_SportPredis"
  preDisMin_TB/1 -> Product15/1
  Add8/1 -> Product15/2
  Constant26/1 -> Add8/1
  [DisplaySpd_kph] -> preDisMin_TB/1, LCS_LC_Emergent_preDis_TB/2
  [Eq_A0] -> LCS_LC_Emergent_preDis_TB/1
  LCS_LC_Emergent_preDis_TB/1 -> Add8/2  "LCS_LC_SportPredisFac"
  Product12/1 -> [Eco_PreDis]  "LCS_LC_EcoPredis"
  LC_Medium_preDis_Fac_TB/1 -> Add7/2  "LCS_LC_EcoPredisFac"
  preDisMin_TB1/1 -> Product12/1
  [Eq_A0] -> LC_Medium_preDis_Fac_TB/1
  [DisplaySpd_kph] -> preDisMin_TB1/1, LC_Medium_preDis_Fac_TB/2
  Constant24/1 -> Add7/1
  Add7/1 -> Product12/2
  Product3/1 -> [Nomal_PreDis]  "LCS_LC_NomalPredis"
  2-D Lookup Table1/1 -> Add5/2  "LCS_LC_NomalPredisFac"
  preDisMin_TB2/1 -> Product3/1  "LCS_Predis_BaseDis"
  Add5/1 -> Product3/2
  Constant22/1 -> Add5/1
  [DisplaySpd_kph] -> preDisMin_TB2/1, 2-D Lookup Table1/2
  TarDangerlLevel2/1 -> Signal Copy6/1
  [Eq_A0] -> 2-D Lookup Table1/1
  Abs1/1 -> [desLaneA0_abs], Divide/1
  [CurrentSteerAngleOffset] -> Saturation/1
  kapTraj1/1 -> [kapTraj]
  desLaneA0_1/1 -> TargetSteerAngleCalc/11(A0)
  [DisplaySpd_kph] -> AngSlopeCalc/2(vDisplay_Kph)
  SteerAngleOffset_deg/1 -> [SteerAngleOffset_deg], Add1/2
  [SteerAngleSpd_degs] -> TargetSteerAngleCalc/13(SteerAngleSpd)
  [LineValid] -> TargetSteerAngleCalc/7(LineValid)
  Constant1/1 -> TargetSteerAngleCalc/6(R1)
  Add6/1 -> Subsystem5/1(raw), Switch1/1, Switch5/3  "LCS_ReqEPSTrgAngle"
  canEPS_LKATorqOvrlDlvd/1 -> [canEPS_LKATorqOvrlDlvd]
  Sum/1 -> [DisplaySpd_kph]  "LCS_DisplaySpd_kph"
  Bias1/1 -> Gain5/1
  Product5/1 -> Add1/1, [LCS_IN_SteerAngle_deg]  "LCS_IN_CurSteerAngle_deg"
  canSteerWheelAngle/1 -> Product5/1
  Gain5/1 -> Product5/2
  [SteerAngle_deg] -> TargetSteerAngleCalc/3(SteerAngle)
  Add1/1 -> [SteerAngle_deg]  "LCS_CurSteerAngle_deg"
  [SteerRatio] -> TargetSteerAngleCalc/4(SteerRatio)
  Gain3/1 -> Gain4/1
  Gain4/1 -> Sum/1
  Constant8/1 -> Sum/2
  [preDis] -> TargetSteerAngleCalc/5(preDis)
  eviVxvRef_ms6/1 -> [vRef], Gain3/1
  TargetSteerAngleCalc/2(LCS_TarSteerAngleEnd) -> Terminator/1  "LCS_TarSteerAngleEnd"
  Signal Copy5/1 -> Abs1/1  "LCS_IN_desLaneA0"
  canSteerWheelAngleSign/1 -> Bias1/1
  TargetSteerAngleCalc/1(TarSteerAngle) -> Add6/1
  Constant/1 -> [SteerRatio]
  eviVxvRef_ms/1 -> TargetSteerAngleCalc/1(vRef)
  [DisplaySpd_kph] -> TargetSteerAngleCalc/2(DisplaySpd_Kph)
  desLaneA2_2/1 -> [desLaneA2]
  canSteerWheelSpd/1 -> Product4/1
  canSteerWheelSpdSign/1 -> Bias2/1
  Gain2/1 -> Product4/2
  Bias2/1 -> Gain2/1
  Product4/1 -> [SteerAngleSpd_degs]  "LCS_IN_SteerAngleSpd_degs"
  desLaneA3/1 -> Signal Copy1/1
  desLaneA1/1 -> Signal Copy3/1
  desLaneA2/1 -> Signal Copy2/1
  TarDangerlLevel/1 -> AngSlopeCalc/1(TarDangerlLevel)
  Saturation/1 -> Add6/2
  [LCS_TarSteerAngleSlope] -> TargetSteerAngleCalc/12("TarSteerAngleSlope ")
  CurrentSteerAngleOffset/1 -> [CurrentSteerAngleOffset]
  Signal Copy/1 -> Direct Lookup Table (n-D)/1  "LCS_IN_TarDangerLevel"
  Saturation1/1 -> TargetSteerAngleCalc/14(CurrentSteerAngleOffset)
  [CurrentSteerAngleOffset] -> Saturation1/1
  [SteerAngleOffset_deg] -> Saturation2/1
  Saturation2/1 -> TargetSteerAngleCalc/15(SteerAngleOffset_deg)
  Data Type Conversion5/1 -> Add3/1
  desLaneA2_3/1 -> Subsystem2/3(desA2), Subsystem/3(desA2)
  PID1/1(Torque) -> Saturation4/1
  desLaneA0_3/1 -> Subsystem2/5(desA0), Subsystem/5(desA0)
  Switch4/1 -> Data Type Conversion5/1  "LCS_ESS_TarAngle"
  [vRef] -> Subsystem2/6(eviVxvRef_ms), Subsystem/6(eviVxvRef_ms1)
  [LineValid] -> Subsystem2/1(desValid), Subsystem/1(desValid)  "Valid"
  desLaneA1_1/1 -> Subsystem2/4(desA1), Subsystem/4(desA1)
  desLaneA3_2/1 -> Subsystem2/2(desA3), Subsystem/2(desA3)
  [kapTraj] -> Subsystem2/8(kap)
  Add/1 -> [AngleError]  "LCS_ControlAngleError"
  Constant5/1 -> Switch4/2
  Saturation4/1 -> Switch2/3  "LCS_ESS_TarTorq"
  Subsystem2/1(LCS_ESS_TarAngle) -> Switch4/3
  [tarAngle] -> Subsystem1/6(tarAngle3)
  Subsystem1/2(TorqValid) -> epsTrqReqFlag/1  "LCS_OUT_EpsTrqReqValueVld"
  Direct Lookup Table (n-D)1/1 -> Compare To Constant/1, Subsystem1/5(<TarDangerLevel>), Subsystem4/8(DangerLevel)
  [SteerAngleFilter_deg] -> Subsystem4/3(curSteerAngle_deg)
  [DisplaySpd_kph] -> Subsystem4/1(VehSpdDisplay)
  [LineValid] -> Subsystem1/4(desLaneValid)  "Valid"
  [isOvride] -> Subsystem4/10(isOvride)
  Subsystem/1(LCS_ESS_TarAngle) -> Switch4/1
  Subsystem4/1(sig_LCKTorq_TorqueCalc) -> Data Type Conversion/1
  Compare To Constant/1 -> Switch2/2  "LCS_DangerLevelisNotESS"
  Product/1 -> Saturation3/1
  [SteerAngleFilter_deg] -> Add3/2
  [Curve] -> Subsystem4/9(Curve)
  Saturation3/1 -> Switch2/1
  canEPS_DrvInputTorq1/1 -> Subsystem4/6(canEPS_DrvInputTorq)
  [SteerAngleSpdFilter_degs] -> Subsystem1/3(SteerAngleSpdWithSign_deg)
  [SteerAngleFilter_deg] -> Subsystem2/7(SteerAngle_deg), Subsystem/7(SteerAngle_deg)
  Add3/1 -> PID1/3(Error)
  [LineValid] -> Subsystem4/7(desLaneValid)  "Valid"
  [SteerAngleSpdFilter_degs] -> Subsystem4/4(canSteerWheelSpd)
  [canEPS_LKATorqOvrlDlvd] -> Subsystem4/5(canEPS_LKATorqOvrlDlvd)
  Switch2/1 -> Subsystem1/1(TorqueCalc)  "LCS_Torq_OUT"
  desLaneA0_4/1 -> Subsystem4/11(Control_A0)
  [SteerAngleFilter_deg] -> Add/2
  Subsystem1/1(TorqueOut) -> epsTrqReqValue/1  "LCS_OUT_EpsTrqReqValue"
  [AngleError] -> Subsystem1/2(AngleError)
  [tarAngle] -> Add/1
  [tarAngle] -> Subsystem4/2(desTarSteerAngle)
  canEPS_DrvInputTorq/1 -> OverRideDetect/1(DrvTrqInput)
  Logical Operator1/1 -> [isOvride]
  OverRideDetect/1(isOverRide) -> Logical Operator1/2  "LCS_IsOverRide"
  Constant15/1 -> Logical Operator1/1
  Signal Copy4/1 -> [LineValid]  "LCS_IN_desLaneValid"
  [TarDangerlLevel] -> Direct Lookup Table (n-D)1/1
  [canEPS_LKATorqOvrlDlvd] -> PID1/2(canEPS_LKATorqOvrlDlvd)
  canEPS_DrvInputTorq2/1 -> PID1/1(canEPS_DrivInputVal)
  [LineValid] -> PID1/4(desLaneValid)
